simulink model "HESS_PID"  (R2020a)
settings: Solver=ode4  StartTime=0.0  StopTime=20  FixedStep=Ts  RelTol=1e-3
PostLoadFcn:
  | Ts =1e-6; load('matlab.mat'); PVMPPT=dato*1150; sizecont5min=size(PVMPPT,1);
InitFcn:
  | Ts =1e-6; load('matlab.mat'); PVMPPT=dato*1150; sizecont5min=size(PVMPPT,1);
values from neighbouring files (symbols this model uses):
  dato = [1.05386503067 1.37609406953 1.24010224949 1.53141104294 1.55073619632 1.53842535787 1.32126789366 1.44051124744 0.80263803681 1.51394683027 1.53785276074 1.45353783231 ... (27 elements, 27x1)]    [matlab.mat]
undefined symbols (not defined in the file or in its folder): DiscIntNeverNeededParam, Ion, Lithium, sizecont
libraries: powerlib x62, powerlib_meascontrol x4, electricdrivelib x1, simulink x1, dspswit3 x1
settings Model: SimulationMode=accelerator  ExplicitPartitioning=on  Creator=Meli  LastModifiedBy=Meli
settings SolverCC: AlgebraicLoopSolver=LineSearch
settings DataIOCC: SaveOutput=off  SaveTime=off  ReturnWorkspaceOutputs=off
settings HardwareCC: ProdHWDeviceType=AMD->x86-64 (Windows64)
settings ModelReferenceCC: ParallelModelReferenceMATLABWorkerInit=Load Top Model
settings RTWCC: BuildConfiguration=Faster Runs
settings CodeAppCC: StateflowObjectComments=on
settings SimscapeCC: SimscapeNormalizeSystem=off

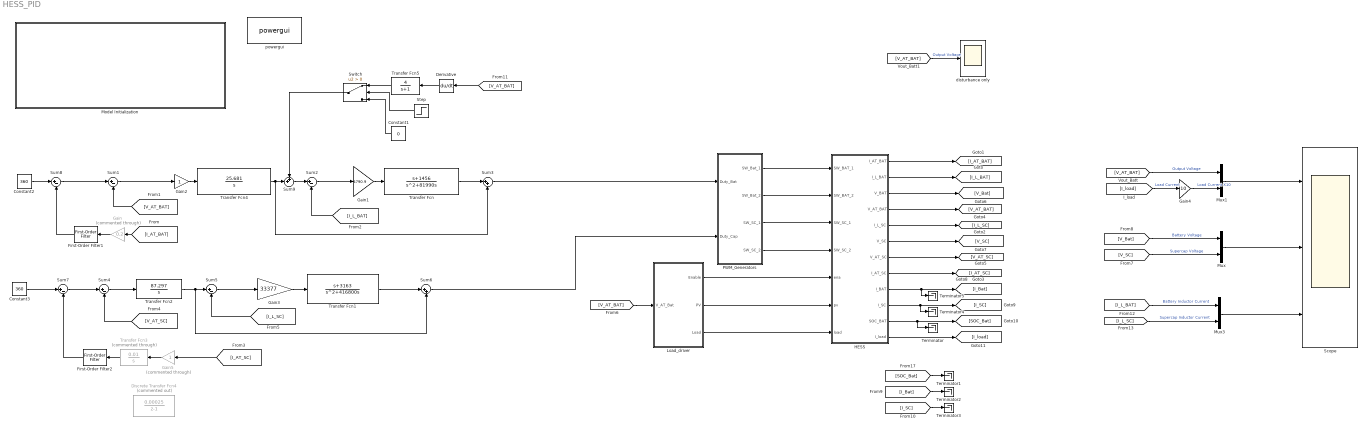
== system HESS_PID ==
  Constant1 : Constant  Value=0
  Constant2 : Constant  Value=360
  Constant3 : Constant  Value=360
  Derivative : Derivative
  Discrete Transfer Fcn4 : DiscreteTransferFcn  Commented=on  Numerator=[0.00025]  Denominator=[1 -1]
  First-Order Filter1 : powerlib_meascontrol/Filters/First-Order Filter  FilterType=Highpass  Tc=1/(2*pi*1)  Ts=0  Initialize=off  Vac_Init=[0, 0, 60]  Vdc_Init=0  PlotResponse=off  FreqRange="[0,  200,  1]"
  First-Order Filter2 : powerlib_meascontrol/Filters/First-Order Filter  FilterType=Lowpass  Tc=1/(2*pi*1)  Ts=0  Initialize=off  Vac_Init=[0, 0, 60]  Vdc_Init=0  PlotResponse=off  FreqRange="[0,  200,  1]"
  Gain : Gain  Commented=through  Gain=0.2
  Gain1 : Gain  Gain=4790.9
  Gain2 : Gain
  Gain3 : Gain  Gain=33377
  Gain4 : Gain  Gain=10
  Gain5 : Gain  Commented=through
  HESS : Subsystem
  Load_driver : Subsystem
  Model Initialization : Subsystem  mask(Model Functions){InitFcnX=Ts =1e-6; load('matlab.mat'); PVMPPT=dato*1150; sizecont5min=size(PVMPPT,1);, prel=off, posl=on, inif=on, strf=off}
      mask prompts: InitFcnX "Initialisation"; prel "Preload Function"; posl "PostLoad Function"; inif "InitFcn"; strf "StartFcn"
      mask init:
      | currentBlock = gcb;
      | root = bdroot(currentBlock);
      | 
      | if ~strcmp(get_param(root,'BlockDiagramType'),'library')
      |     if prel==1
      |         set_param(root, 'PreLoadFcn', InitFcnX);
      |     else
      |         set_param(root, 'PreLoadFcn', '');
      |     end
      |     if inif==1
      |         set_param(root, 'InitFcn', InitFcnX);
      |     else
      |         set_param(root, 'InitFcn', '');
      |     end
      |     if strf==1
      |         set_param(root, 'StartFcn', InitFcnX);
      |     else
      |         set_param(root, 'StartFcn', '');
      |     end
      |     if posl==1
      |         set_param(root, 'PostLoadFcn', InitFcnX);
      |     else
      |         set_param(root, 'PostLoadFcn', '');
      |     end
      | end
      | 
      | pos = get_param(currentBlock, 'Position');
      | width = pos(3) - pos(1); height = pos(4) - pos(2);
      | txt = [ upper(root) '\n' '- InitFcn. . . . . '  get_param(root, 'InitFcn') ];
      settings: CopyFcn=set_param(gcb,'LinkStatus','none')
      mask Display: text(5, height*0.5, txt, 'horizontalAlignment', 'left', 'verticalAlignment', 'middle') ;
  Mux : Mux  Inputs=2
  Mux1 : Mux  Inputs=2
  Mux3 : Mux  Inputs=2
  PWM_Generators : Subsystem
  Scope : Scope  NumInputPorts=3
  Step : Step  Time=10  SampleTime=0
  Sum{1..2,4..5,7..8} (6 alike) : Sum  Inputs=|+-
  Sum3 : Sum  Inputs=|++
  Sum6 : Sum  Inputs=|++
  Sum9 : Sum  Inputs=++|
  Switch : Switch  Criteria=u2 > Threshold
  Terminator{,1..5} (6 alike) : Terminator
  Transfer Fcn : TransferFcn  Numerator=[1 1456]  Denominator=[1 81990 0]
  Transfer Fcn1 : TransferFcn  Numerator=[1 3163]  Denominator=[1 416800 0]
  Transfer Fcn2 : TransferFcn  Numerator=[87.297]  Denominator=[1 0]
  Transfer Fcn3 : TransferFcn  Commented=through  Numerator=[0.01]  Denominator=[1 0]
  Transfer Fcn4 : TransferFcn  Numerator=[25.681]  Denominator=[1 0]
  Transfer Fcn5 : TransferFcn  Numerator=[4]  Denominator=[1 1]
  disturbance only : Scope
  powergui : powerlib/powergui  Priority=1  SimulationMode=Discrete  SampleTime=Ts  frequency=60  Iterations=50  frequencyindice=0  Pbase=100e6  ErrMax=1e-4  UnitsV=kV  UnitsW=MW  buscounter=0  FunctionMessages=off  echomessages=off  EnableUseOfTLC=off  CurrentSourceSwitches=off  DisableSnubberDevices=off  DisableRonSwitches=off  DisableVfSwitches=off  DisplayEquations=off  AutomaticDiscreteSolvers=off  SolverType=Tustin/Backward Euler (TBE)  Interpol=off  ExternalGateDelay=off  methode=off  Ts=100  x0status=blocks  SPID=on  SwTol=0  HookPort=off  NonlinearTolerance=1e-4  nMaxIteration=100  ContinueOnMaxIteration=off  RestoreLinks=warning  ResistiveCurrentMeasurement=off  Frange=[0:2:500]  Ylog=off  Xlog=on  ShowGrid=off  save=off  variable=ZData  structure=ScopeData  ZoomFFT=off  StartTime=7.29  cycles=3  DisplayStyle=1  fundamental=50  FreqAxis=off  MaxFrequency=1000  frequencyindicesteady=1  RmsSteady=1  display=off
  wires:
  PWM_Generators/1(SW_Bat_1) -> HESS/1(SW_BAT_1)
  PWM_Generators/2(SW_Bat_2) -> HESS/2(SW_BAT_2)
  PWM_Generators/3(SW_SC_1) -> HESS/3(SW_SC_1)
  PWM_Generators/4(SW_SC_2) -> HESS/4(SW_SC_2)
  Sum2/1 -> Gain1/1
  Gain/1 -> First-Order Filter1/1
  Gain2/1 -> Transfer Fcn4/1
  Transfer Fcn/1 -> Sum3/1
  [V_AT_BAT] -> Sum1/2
  Gain1/1 -> Transfer Fcn/1
  Sum3/1 -> PWM_Generators/1(Duty_Bat)
  Sum1/1 -> Gain2/1
  [I_AT_BAT] -> Gain/1
  [I_L_BAT] -> Sum2/2
  Sum8/1 -> Sum1/1
  Constant2/1 -> Sum8/1
  Gain5/1 -> Transfer Fcn3/1
  [I_L_SC] -> Sum5/2
  Sum4/1 -> Transfer Fcn2/1
  [V_AT_SC] -> Sum4/2
  Gain3/1 -> Transfer Fcn1/1
  [I_AT_SC] -> Gain5/1
  Transfer Fcn2/1 -> Sum6/2, Sum5/1
  Sum5/1 -> Gain3/1
  Transfer Fcn3/1 -> First-Order Filter2/1
  Transfer Fcn1/1 -> Sum6/1
  Sum7/1 -> Sum4/1
  Constant3/1 -> Sum7/1
  Sum6/1 -> PWM_Generators/2(Duty_Cap)
  HESS/1(I_AT_BAT) -> [I_AT_BAT]
  HESS/2(I_L_BAT) -> [I_L_BAT]
  HESS/5(I_L_SC) -> [I_L_SC]
  HESS/8(I_AT_SC) -> [I_AT_SC]
  HESS/7(V_AT_SC) -> [V_AT_SC]
  HESS/4(V_AT_BAT) -> [V_AT_BAT]
  Load_driver/1(Enable) -> HESS/5(ena)
  Load_driver/2(PV) -> HESS/6(pv)
  Load_driver/3(Load) -> HESS/7(load)
  [V_AT_BAT] -> Load_driver/1(V_AT_Bat)
  HESS/3(V_BAT) -> [V_Bat]
  HESS/6(V_SC) -> [V_SC]
  HESS/9(I_BAT) -> Terminator5/1, [I_Bat]
  HESS/10(I_SC) -> Terminator4/1, [I_SC]
  HESS/11(SOC_BAT) -> Terminator/1, [SOC_Bat]
  HESS/12(I_load) -> [I_load]
  [V_Bat] -> Mux/1  "Battery Voltage"
  [V_SC] -> Mux/2  "Supercap Voltage"
  [V_AT_BAT] -> Mux1/1  "Output Voltage"
  [SOC_Bat] -> Terminator1/1
  [I_load] -> Gain4/1  "Load Current"
  [I_L_BAT] -> Mux3/1  "Battery Inductor Current"
  [I_L_SC] -> Mux3/2  "Supercap Inductor Current"
  [I_Bat] -> Terminator2/1
  [I_SC] -> Terminator3/1
  Mux1/1 -> Scope/1
  Mux/1 -> Scope/2
  Mux3/1 -> Scope/3
  First-Order Filter1/1 -> Sum8/2
  First-Order Filter2/1 -> Sum7/2
  Gain4/1 -> Mux1/2  "Load Current X10"
  Sum9/1 -> Sum2/1
  Transfer Fcn4/1 -> Sum3/2, Sum9/2
  Derivative/1 -> Transfer Fcn5/1
  [V_AT_BAT] -> Derivative/1
  [V_AT_BAT] -> disturbance only/1  "Output Voltage"
  Transfer Fcn5/1 -> Switch/1
  Switch/1 -> Sum9/1
  Step/1 -> Switch/2
  Constant1/1 -> Switch/3

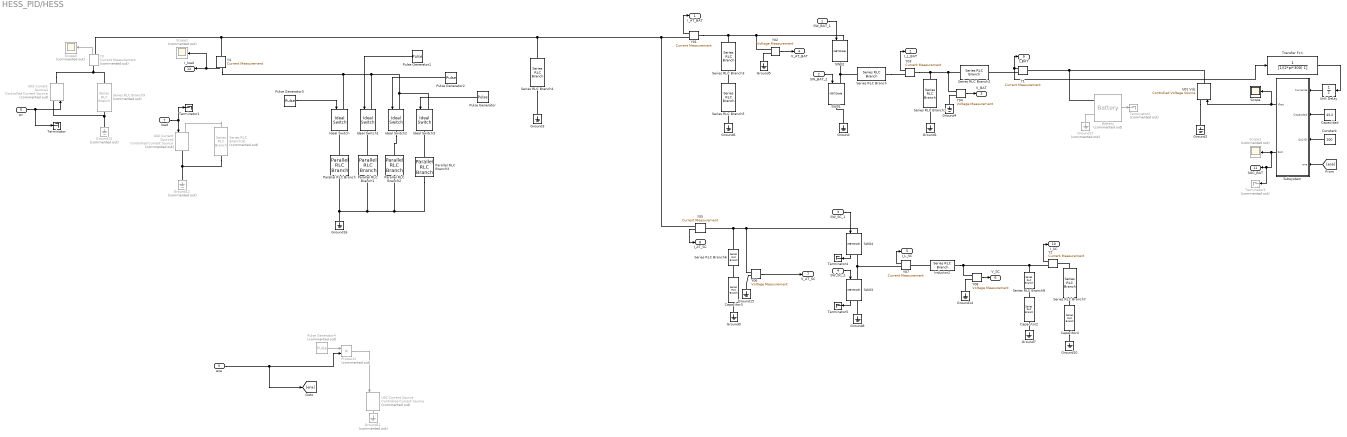
== system HESS_PID/HESS ==
  SW_BAT_1 : Inport
  SW_BAT_2 : Inport  Port=2
  SW_SC_1 : Inport  Port=3
  SW_SC_2 : Inport  Port=4
  ena : Inport  Port=5
  pv : Inport  Port=6
  load : Inport  Port=7
  Battery : electricdrivelib/Extra Sources/Battery  Commented=on  BatType=Lithium-Ion  ShowTempParam=off  ThermalPreset="12.8V  40Ah  (LiFeMgPO4)"  ShowAgeParam=off  NomV=144  NomQ=43.2  SOC=80  Batt_Tr=5  PresetModel=on  MaxQ=43.2  MinV=108  FullV=167.6141  Dis_rate=18.7826  R=0.033333  Normal_OP=39.0678  expZone="[155.5756      2.122435]"  current=[2.3 4.5 6 10]  Units=Time  Tci=20  NomT=20  T2=0  MaxQ2=36  FullV2=13  Normal_OP2=11.7  expZone2="[12.67            4]"  Rca=0.6411  ti=4880  Dp=0  Neq0=0  Tsim=1e6  Ta1=25  Qeol=5.4*0.9  Reol=0.013333*1.2  Char_age=[2.3478, 3]  Dis_age=[2.3478, 10]  N1=1500  N2=10500  N3=1000  N4=1400  Ta2=45  N5=950
  Capacidad : Constant  Value=43.2
  Capacitor2 : powerlib/Elements/Series RLC Branch  LConnTagsString=__new0  RConnTagsString=__new0  BranchType=C  Resistance=1  Inductance=1e-3  SetiL0=off  InitialCurrent=0  Capacitance=390e-6  Setx0=on  InitialVoltage=189  Measurements=None
  Capacitor3 : powerlib/Elements/Series RLC Branch  LConnTagsString=__new0  RConnTagsString=__new0  BranchType=C  Resistance=1  Inductance=1e-3  SetiL0=off  InitialCurrent=0  Capacitance=1.29e-3  Setx0=on  InitialVoltage=360  Measurements=None
  Capacitor4 : powerlib/Elements/Series RLC Branch  LConnTagsString=__new0  RConnTagsString=__new0  BranchType=C  Resistance=1  Inductance=1e-3  SetiL0=off  InitialCurrent=0  Capacitance=20  Setx0=on  InitialVoltage=189.34  Measurements=None
  Constant : Constant  Value=100
  Ground{,1..10,14..16} (14 alike) : powerlib/Elements/Ground  LConnTagsString=a
  Ground{11..13,17} (4 alike) : powerlib/Elements/Ground  Commented=on  LConnTagsString=a
  Ideal Switch{,1..3} (4 alike) : powerlib/Power Electronics/Ideal Switch  Ron=1e-6  Lon=0  IC=0  Rs=inf  Cs=0  Measurements=off
  Inductor2 : powerlib/Elements/Series RLC Branch  LConnTagsString=__new0  RConnTagsString=__new0  BranchType=L  Resistance=1  Inductance=4.6e-3  SetiL0=off  InitialCurrent=0  Capacitance=1e-6  Setx0=off  InitialVoltage=0  Measurements=None
  Parallel RLC Branch : powerlib/Elements/Parallel RLC Branch  LConnTagsString=a  RConnTagsString=__new0  BranchType=R  Resistance=109.14  Inductance=1e-9  SetiL0=off  InitialCurrent=0  Capacitance=1e-6  Setx0=off  InitialVoltage=0  Measurements=None
  Parallel RLC Branch1 : powerlib/Elements/Parallel RLC Branch  LConnTagsString=a  RConnTagsString=__new0  BranchType=R  Resistance=109.14  Inductance=1e-3  SetiL0=off  InitialCurrent=0  Capacitance=1e-6  Setx0=off  InitialVoltage=0  Measurements=None
  Parallel RLC Branch2 : powerlib/Elements/Parallel RLC Branch  LConnTagsString=a  RConnTagsString=__new0  BranchType=R  Resistance=109.14  Inductance=1e-3  SetiL0=off  InitialCurrent=0  Capacitance=1e-6  Setx0=off  InitialVoltage=0  Measurements=None
  Parallel RLC Branch3 : powerlib/Elements/Parallel RLC Branch  LConnTagsString=a  RConnTagsString=__new0  BranchType=R  Resistance=109.14  Inductance=1e-3  SetiL0=off  InitialCurrent=0  Capacitance=1e-6  Setx0=off  InitialVoltage=0  Measurements=None
  Product1 : Product  Commented=on
  Pulse Generator : DiscretePulseGenerator  PulseType=Time based  Amplitude=4  Period=6  PulseWidth=8.335  PhaseDelay=5.5
  Pulse Generator1 : DiscretePulseGenerator  PulseType=Time based  Amplitude=2  PulseWidth=50  PhaseDelay=2
  Pulse Generator2 : DiscretePulseGenerator  PulseType=Time based  Amplitude=3  Period=6  PulseWidth=16.667  PhaseDelay=2.5
  Pulse Generator3 : DiscretePulseGenerator  PulseType=Time based  Amplitude=2  Period=13  PulseWidth=50  PhaseDelay=0.2
  Pulse Generator4 : DiscretePulseGenerator  Commented=on  PulseType=Time based  Amplitude=5.4  Period=0.2  PulseWidth=30  PhaseDelay=0.2
  SW01 : powerlib/Power Electronics/IGBT//Diode  Ron=1e-3  Rs=1e5  Cs=inf  Measurements=off
  SW02 : powerlib/Power Electronics/IGBT//Diode  Ron=1e-3  Rs=Inf  Cs=inf  Measurements=off
  SW03 : powerlib/Power Electronics/IGBT//Diode  Ron=1e-6  Rs=1e8  Cs=inf  Measurements=on
  SW04 : powerlib/Power Electronics/IGBT//Diode  Ron=1e-6  Rs=1e8  Cs=inf  Measurements=on
  Scope : Scope
  Scope1 : Scope  Commented=on
  Scope2 : Scope  Commented=on
  Scope3 : Scope  Commented=on
  Series RLC Branch : powerlib/Elements/Series RLC Branch  LConnTagsString=__new0  RConnTagsString=__new0  BranchType=L  Resistance=1  Inductance=5.2e-3  SetiL0=off  InitialCurrent=0  Capacitance=1e-6  Setx0=off  InitialVoltage=0  Measurements=None
  Series RLC Branch1 : powerlib/Elements/Series RLC Branch  LConnTagsString=__new0  RConnTagsString=__new0  BranchType=C  Resistance=1  Inductance=100e-3  SetiL0=off  InitialCurrent=0  Capacitance=100e-3  Setx0=on  InitialVoltage=144  Measurements=None
  Series RLC Branch10 : powerlib/Elements/Series RLC Branch  Commented=on  LConnTagsString=__new0  RConnTagsString=__new0  BranchType=R  Resistance=10000000000  Inductance=6e-3  SetiL0=off  InitialCurrent=0  Capacitance=1e-6  Setx0=off  InitialVoltage=0  Measurements=None
  Series RLC Branch2 : powerlib/Elements/Series RLC Branch  LConnTagsString=__new0  RConnTagsString=__new0  BranchType=R  Resistance=100e-3  Inductance=6e-3  SetiL0=off  InitialCurrent=0  Capacitance=1e-6  Setx0=off  InitialVoltage=0  Measurements=None
  Series RLC Branch3 : powerlib/Elements/Series RLC Branch  LConnTagsString=__new0  RConnTagsString=__new0  BranchType=R  Resistance=1e-3  Inductance=6e-3  SetiL0=off  InitialCurrent=0  Capacitance=1e-6  Setx0=off  InitialVoltage=0  Measurements=None
  Series RLC Branch4 : powerlib/Elements/Series RLC Branch  LConnTagsString=__new0  RConnTagsString=__new0  BranchType=R  Resistance=560  Inductance=6e-3  SetiL0=off  InitialCurrent=0  Capacitance=1e-6  Setx0=off  InitialVoltage=0  Measurements=None
  Series RLC Branch5 : powerlib/Elements/Series RLC Branch  LConnTagsString=__new0  RConnTagsString=__new0  BranchType=C  Resistance=1  Inductance=100e-3  SetiL0=off  InitialCurrent=0  Capacitance=2.6267e-4  Setx0=on  InitialVoltage=360  Measurements=None
  Series RLC Branch6 : powerlib/Elements/Series RLC Branch  LConnTagsString=__new0  RConnTagsString=__new0  BranchType=R  Resistance=1e-3  Inductance=0  SetiL0=off  InitialCurrent=0  Capacitance=0  Setx0=off  InitialVoltage=0  Measurements=None
  Series RLC Branch7 : powerlib/Elements/Series RLC Branch  LConnTagsString=__new0  RConnTagsString=__new0  BranchType=R  Resistance=0.3405  Inductance=0  SetiL0=off  InitialCurrent=0  Capacitance=0  Setx0=off  InitialVoltage=0  Measurements=None
  Series RLC Branch8 : powerlib/Elements/Series RLC Branch  LConnTagsString=__new0  RConnTagsString=__new0  BranchType=R  Resistance=1e-3  Inductance=0  SetiL0=off  InitialCurrent=0  Capacitance=0  Setx0=off  InitialVoltage=0  Measurements=None
  Series RLC Branch9 : powerlib/Elements/Series RLC Branch  Commented=on  LConnTagsString=__new0  RConnTagsString=__new0  BranchType=R  Resistance=10000000000  Inductance=6e-3  SetiL0=off  InitialCurrent=0  Capacitance=1e-6  Setx0=off  InitialVoltage=0  Measurements=None
  Subsystem : Subsystem
  Terminator{,1,4..5} (4 alike) : Terminator
  Terminator2 : Terminator  Commented=on
  Terminator3 : Terminator  Commented=on
  Transfer Fcn : TransferFcn  Denominator=[1/(2*pi*300) 1]
  U01 Vdc : powerlib/Electrical Sources/Controlled Voltage Source  Initialize=on  Source_Type=DC  Amplitude=144  Phase=0  Frequency=0  Measurements=None
  U02 Current Source : powerlib/Electrical Sources/Controlled Current Source  Commented=on  Initialize=on  Source_Type=AC  Amplitude=0  Phase=0  Frequency=0  Measurements=None
  U02 Current Source1 : powerlib/Electrical Sources/Controlled Current Source  Commented=on  Initialize=on  Source_Type=DC  Amplitude=0  Phase=0  Frequency=0  Measurements=None
  U02 Current Source2 : powerlib/Electrical Sources/Controlled Current Source  Commented=on  Initialize=on  Source_Type=DC  Amplitude=0  Phase=0  Frequency=0  Measurements=None
  Unit Delay : UnitDelay  SampleTime=Ts  HasFrameUpgradeWarning=on
  Y01 : powerlib/Measurements/Current Measurement  PhasorSimulation=off  OutputType=Complex  PSBequivalent=0
  Y02 : powerlib/Measurements/Voltage Measurement  PhasorSimulation=off  OutputType=Complex  PSBequivalent=0
  Y03 : powerlib/Measurements/Current Measurement  PhasorSimulation=off  OutputType=Complex  PSBequivalent=0
  Y04 : powerlib/Measurements/Voltage Measurement  PhasorSimulation=off  OutputType=Complex  PSBequivalent=0
  Y05 : powerlib/Measurements/Current Measurement  PhasorSimulation=off  OutputType=Complex  PSBequivalent=0
  Y06 : powerlib/Measurements/Voltage Measurement  PhasorSimulation=off  OutputType=Complex  PSBequivalent=0
  Y07 : powerlib/Measurements/Current Measurement  PhasorSimulation=off  OutputType=Complex  PSBequivalent=0
  Y08 : powerlib/Measurements/Voltage Measurement  PhasorSimulation=off  OutputType=Complex  PSBequivalent=0
  Y1 : powerlib/Measurements/Current Measurement  PhasorSimulation=off  OutputType=Complex  PSBequivalent=0
  Y2 : powerlib/Measurements/Current Measurement  PhasorSimulation=off  OutputType=Complex  PSBequivalent=0
  Y3 : powerlib/Measurements/Current Measurement  Commented=on  PhasorSimulation=off  OutputType=Complex  PSBequivalent=0
  Y4 : powerlib/Measurements/Current Measurement  PhasorSimulation=off  OutputType=Complex  PSBequivalent=0
  I_AT_BAT : Outport
  I_L_BAT : Outport  Port=2
  V_BAT : Outport  Port=3
  V_AT_BAT : Outport  Port=4
  I_L_SC : Outport  Port=5
  V_SC : Outport  Port=6
  V_AT_SC : Outport  Port=7
  I_AT_SC : Outport  Port=8
  I_BAT : Outport  Port=9
  I_SC : Outport  Port=10
  SOC_BAT : Outport  Port=11
  I_load : Outport  Port=12
  wires:
  SW04/1 -> Terminator4/1
  Y08/1 -> V_SC/1
  [ena] -> Subsystem/4(ena)
  Subsystem/1(Vbat) -> Scope/1, U01 Vdc/1
  Subsystem/2(SoC) -> Terminator3/1, SOC_BAT/1, Scope1/1
  SW_SC_1/1 -> SW04/1
  Y01/1 -> I_AT_BAT/1
  Y07/1 -> I_L_SC/1
  Pulse Generator4/1 -> Product1/1
  SW_BAT_2/1 -> SW01/1
  SW03/1 -> Terminator5/1
  Y2/1 -> I_SC/1
  Y04/1 -> V_BAT/1
  pv/1 -> Terminator/1, U02 Current Source1/1
  load/1 -> Terminator1/1, U02 Current Source2/1
  Y05/1 -> I_AT_SC/1
  ena/1 -> [ena], Product1/2
  Y03/1 -> I_L_BAT/1
  Product1/1 -> U02 Current Source/1
  SW_SC_2/1 -> SW03/1
  Unit Delay/1 -> Subsystem/1(Corriente)
  Constant/1 -> Subsystem/3(SoC(0))
  Y1/1 -> I_BAT/1, Transfer Fcn/1
  Y02/1 -> V_AT_BAT/1
  Y3/1 -> Scope3/1
  SW_BAT_1/1 -> SW02/1
  Capacidad/1 -> Subsystem/2(Capacidad)
  Y06/1 -> V_AT_SC/1
  Transfer Fcn/1 -> Unit Delay/1
  Pulse Generator2/1 -> Ideal Switch2/1
  Pulse Generator/1 -> Ideal Switch3/1
  Pulse Generator3/1 -> Ideal Switch/1
  Pulse Generator1/1 -> Ideal Switch1/1
  Battery/1 -> Terminator2/1
  Y4/1 -> Scope2/1, I_load/1
  connections:
  U02 Current Source2/RConn1 -- Series RLC Branch10/RConn1 -- Ground12/LConn1
  U02 Current Source1/LConn1 -- Series RLC Branch9/RConn1 -- Ground13/LConn1
  Series RLC Branch10/LConn1 -- U02 Current Source2/LConn1
  U02 Current Source1/RConn1 -- Series RLC Branch9/LConn1 -- Y3/LConn1
  SW02/LConn1 -- Y02/LConn1 -- Series RLC Branch3/LConn1 -- Y01/LConn1
  SW04/RConn1 -- SW03/LConn1 -- Y07/RConn1
  Y04/LConn1 -- Series RLC Branch2/LConn1 -- Y03/LConn1 -- Series RLC Branch1/LConn1
  Series RLC Branch8/LConn1 -- Y2/RConn1 -- Y08/LConn1 -- Inductor2/RConn1
  Y05/RConn1 -- Y01/RConn1 -- Y3/RConn1 -- Y4/LConn1 -- Series RLC Branch4/LConn1
  Y06/LConn1 -- SW04/LConn1 -- Series RLC Branch6/LConn1 -- Y05/LConn1
  SW02/RConn1 -- Series RLC Branch/LConn1 -- SW01/LConn1
  Capacitor3/LConn1 -- Series RLC Branch6/RConn1
  Ground8/LConn1 -- SW03/RConn1
  Ground/LConn1 -- SW01/RConn1
  Series RLC Branch/RConn1 -- Y03/RConn1
  Ground5/LConn1 -- Y02/LConn2
  Series RLC Branch7/LConn1 -- Y2/LConn1
  Series RLC Branch5/LConn1 -- Series RLC Branch3/RConn1
  Ground7/LConn1 -- Capacitor2/RConn1
  Series RLC Branch4/RConn1 -- Ground3/LConn1
  Inductor2/LConn1 -- Y07/LConn1
  U01 Vdc/RConn1 -- Battery/LConn1 -- Y1/LConn1
  Capacitor2/LConn1 -- Series RLC Branch8/RConn1
  Ground9/LConn1 -- Capacitor3/RConn1
  Ground15/LConn1 -- Y06/LConn2
  Ground6/LConn1 -- Series RLC Branch5/RConn1
  Ground1/LConn1 -- Series RLC Branch1/RConn1
  U01 Vdc/LConn1 -- Ground2/LConn1
  Capacitor4/LConn1 -- Series RLC Branch7/RConn1
  Y1/RConn1 -- Series RLC Branch2/RConn1
  Ground4/LConn1 -- Y04/LConn2
  Capacitor4/RConn1 -- Ground10/LConn1
  Ground11/LConn1 -- U02 Current Source/RConn1
  Y08/LConn2 -- Ground14/LConn1
  Parallel RLC Branch2/RConn1 -- Ground16/LConn1 -- Parallel RLC Branch/RConn1 -- Parallel RLC Branch1/RConn1 -- Parallel RLC Branch3/RConn1
  Ideal Switch1/LConn1 -- Ideal Switch3/LConn1 -- Ideal Switch2/LConn1 -- Y4/RConn1 -- Ideal Switch/LConn1
  Parallel RLC Branch/LConn1 -- Ideal Switch/RConn1
  Parallel RLC Branch3/LConn1 -- Ideal Switch3/RConn1
  Parallel RLC Branch1/LConn1 -- Ideal Switch1/RConn1
  Ideal Switch2/RConn1 -- Parallel RLC Branch2/LConn1
  Battery/LConn2 -- Ground17/LConn1

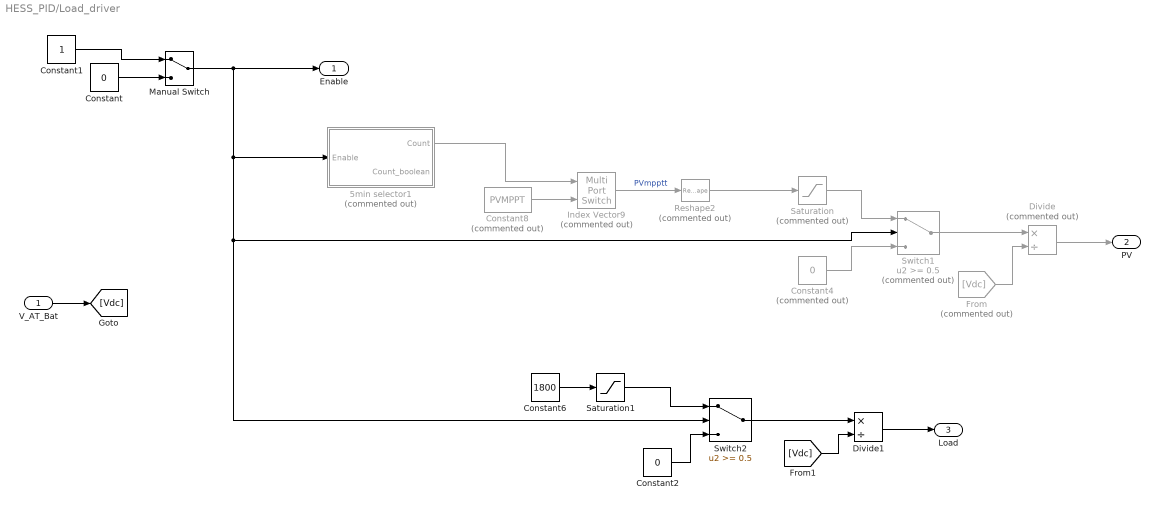
== system HESS_PID/Load_driver ==
  V_AT_Bat : Inport
  5min selector1 : Subsystem  Commented=on
  Constant : Constant  Value=0
  Constant1 : Constant
  Constant2 : Constant  Value=0
  Constant4 : Constant  Commented=on  Value=0
  Constant6 : Constant  Value=1800
  Constant8 : Constant  Commented=on  Value=PVMPPT
  Divide : Product  Commented=on  Inputs=*/
  Divide1 : Product  Inputs=*/
  From : From  Commented=on  GotoTag=Vdc
  Index Vector9 : MultiPortSwitch  Commented=on  DataPortOrder=Zero-based contiguous  Inputs=1  zeroidx=on
  Manual Switch : ManualSwitch
  Reshape2 : Reshape  Commented=on  OutputDimensionality=Customize  OutputDimensions=[1]
  Saturation : Saturate  Commented=on  UpperLimit=4000  LowerLimit=0
  Saturation1 : Saturate  UpperLimit=5000  LowerLimit=0
  Switch1 : Switch  Commented=on  Threshold=0.5
  Switch2 : Switch  Threshold=0.5
  Enable : Outport
  PV : Outport  Port=2
  Load : Outport  Port=3
  wires:
  Reshape2/1 -> Saturation/1
  Saturation/1 -> Switch1/1
  Index Vector9/1 -> Reshape2/1  "PVmpptt"
  From/1 -> Divide/2
  Constant/1 -> Manual Switch/2
  Constant6/1 -> Saturation1/1
  5min selector1/1(Count) -> Index Vector9/1
  Constant8/1 -> Index Vector9/2
  Manual Switch/1 -> 5min selector1/1(Enable), Switch2/2, Switch1/2, Enable/1
  Divide/1 -> PV/1
  Divide1/1 -> Load/1
  Constant2/1 -> Switch2/3
  [Vdc] -> Divide1/2
  Switch2/1 -> Divide1/1
  Constant4/1 -> Switch1/3
  Switch1/1 -> Divide/1
  Constant1/1 -> Manual Switch/1
  Saturation1/1 -> Switch2/1
  V_AT_Bat/1 -> [Vdc]

== system HESS_PID/Model Initialization ==

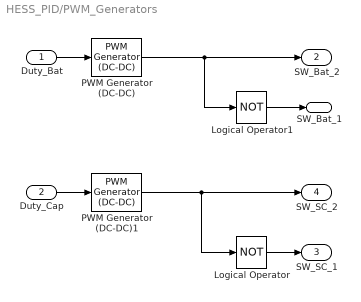
== system HESS_PID/PWM_Generators ==
  Duty_Bat : Inport
  Duty_Cap : Inport  Port=2
  Logical Operator : Logic  Operator=NOT  AllPortsSameDT=off  OutDataTypeStr=boolean
  Logical Operator1 : Logic  Operator=NOT  AllPortsSameDT=off  OutDataTypeStr=boolean
  PWM Generator (DC-DC) : powerlib_meascontrol/Pulse & Signal Generators/PWM Generator (DC-DC)  Fsw=10000  Ts=Ts
  PWM Generator (DC-DC)1 : powerlib_meascontrol/Pulse & Signal Generators/PWM Generator (DC-DC)  Fsw=30000  Ts=Ts
  SW_Bat_1 : Outport
  SW_Bat_2 : Outport  Port=2
  SW_SC_1 : Outport  Port=3
  SW_SC_2 : Outport  Port=4
  wires:
  Duty_Cap/1 -> PWM Generator (DC-DC)1/1
  Duty_Bat/1 -> PWM Generator (DC-DC)/1
  PWM Generator (DC-DC)/1 -> Logical Operator1/1, SW_Bat_2/1
  PWM Generator (DC-DC)1/1 -> SW_SC_2/1, Logical Operator/1
  Logical Operator/1 -> SW_SC_1/1
  Logical Operator1/1 -> SW_Bat_1/1

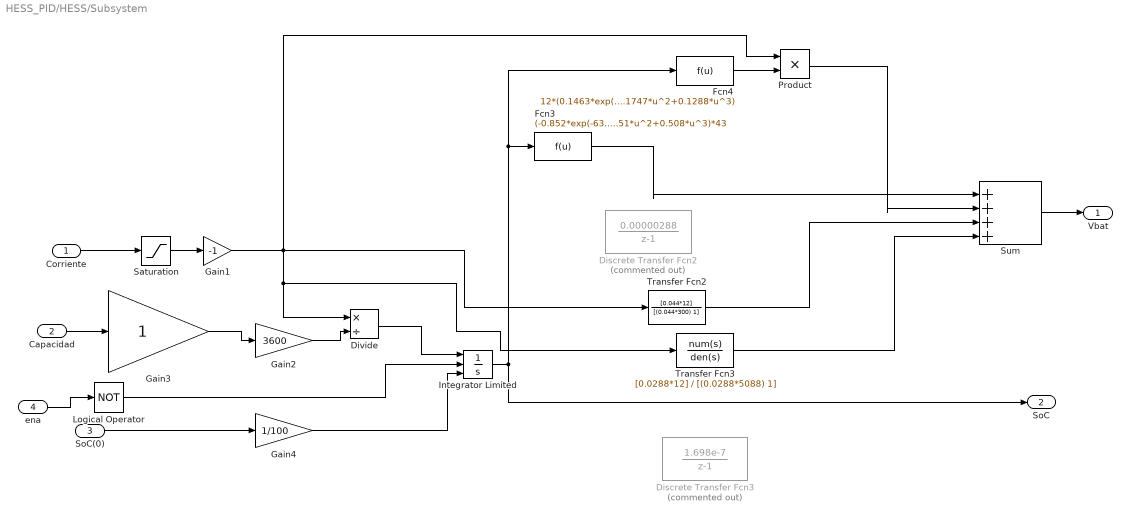
== system HESS_PID/HESS/Subsystem ==
  Corriente : Inport
  Capacidad : Inport  Port=2
  SoC(0) : Inport  Port=3
  ena : Inport  Port=4
  Discrete Transfer Fcn2 : DiscreteTransferFcn  Commented=on  Numerator=[0.00000288]  Denominator=[1 -1]
  Discrete Transfer Fcn3 : DiscreteTransferFcn  Commented=on  Numerator=[1.698e-7]  Denominator=[1 -1]
  Divide : Product  Inputs=*/
  Fcn3 : Fcn  Expr=(-0.852*exp(-63.867*u)+3.6297+0.559*u-0.51*u^2+0.508*u^3)*43
  Fcn4 : Fcn  Expr=12*(0.1463*exp(-30.27*u)+0.1037+0.0584*u-0.1747*u^2+0.1288*u^3)
  Gain1 : Gain  Gain=-1
  Gain2 : Gain  Gain=3600
  Gain3 : Gain
  Gain4 : Gain  Gain=1/100
  Integrator Limited : Integrator  ExternalReset=level  InitialConditionSource=external  LimitOutput=on  UpperSaturationLimit=1.2  LowerSaturationLimit=0
  Logical Operator : Logic  Operator=NOT  AllPortsSameDT=off  OutDataTypeStr=boolean
  Product : Product
  Saturation : Saturate  UpperLimit=20  LowerLimit=-20
  Sum : Sum  Inputs=|++++
  Transfer Fcn2 : TransferFcn  Numerator=[0.044*12]  Denominator=[(0.044*300) 1]
  Transfer Fcn3 : TransferFcn  Numerator=[0.0288*12]  Denominator=[(0.0288*5088) 1]
  Vbat : Outport
  SoC : Outport  Port=2
  wires:
  Gain1/1 -> Transfer Fcn2/1, Product/1, Transfer Fcn3/1, Divide/1
  Fcn3/1 -> Sum/1
  Product/1 -> Sum/2
  Fcn4/1 -> Product/2
  Gain3/1 -> Gain2/1
  Transfer Fcn2/1 -> Sum/3
  Logical Operator/1 -> Integrator Limited/2
  Capacidad/1 -> Gain3/1
  Integrator Limited/1 -> SoC/1, Fcn3/1, Fcn4/1
  SoC(0)/1 -> Gain4/1
  Transfer Fcn3/1 -> Sum/4
  Gain4/1 -> Integrator Limited/3
  Divide/1 -> Integrator Limited/1
  Gain2/1 -> Divide/2
  Corriente/1 -> Saturation/1
  Sum/1 -> Vbat/1
  ena/1 -> Logical Operator/1
  Saturation/1 -> Gain1/1

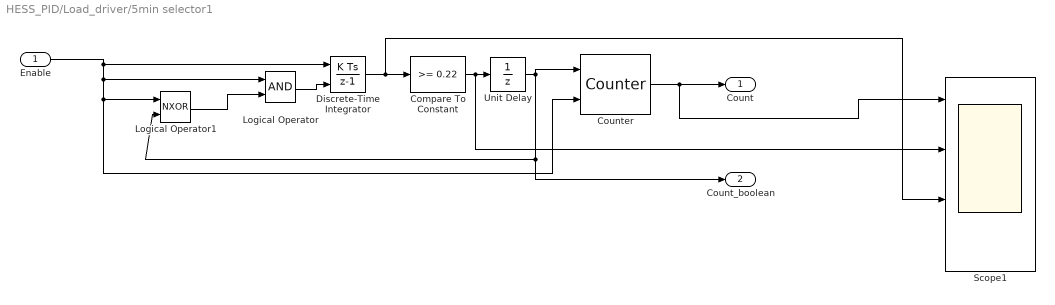
== system HESS_PID/Load_driver/5min selector1 ==
  Enable : Inport
  Compare To Constant : simulink/Logic and Bit Operations/Compare To Constant  relop=>=  const=0.22  OutDataTypeStr=boolean
  Counter : dspswit3/Counter  Direction=Up  CountEvent=Rising edge  CounterSize=User defined  MaxCount=sizecont5min-1  InitialCount=0  Output=Count  HitValue=sizecont-1  ResetInput=on  SamplesPerFrame=1  Ts=1  CntDtype=double  HitDtype=Logical
  Discrete-Time Integrator : DiscreteIntegrator  ExternalReset=rising  SampleTime=Ts  ICPrevOutput=DiscIntNeverNeededParam  ICPrevScaledInput=DiscIntNeverNeededParam
  Logical Operator : Logic  AllPortsSameDT=off  OutDataTypeStr=boolean
  Logical Operator1 : Logic  Operator=NXOR  AllPortsSameDT=off  OutDataTypeStr=boolean
  Scope1 : Scope  NumInputPorts=4
  Unit Delay : UnitDelay  SampleTime=-1  HasFrameUpgradeWarning=on
  Count : Outport
  Count_boolean : Outport  Port=2
  wires:
  Logical Operator/1 -> Discrete-Time Integrator/2
  Unit Delay/1 -> Counter/1, Count_boolean/1, Logical Operator1/2
  Enable/1 -> Counter/2, Logical Operator1/1, Logical Operator/1, Discrete-Time Integrator/1
  Discrete-Time Integrator/1 -> Scope1/3, Compare To Constant/1
  Compare To Constant/1 -> Scope1/2, Unit Delay/1
  Logical Operator1/1 -> Logical Operator/2
  Counter/1 -> Scope1/1, Count/1
